simulink model "turbina_viento"  (R2015a)
settings: Solver=ode45  StartTime=0.0  StopTime=50  RelTol=1e-3
libraries: simulink x1
settings Model: Creator=Administrador  LastModifiedBy=Administrador

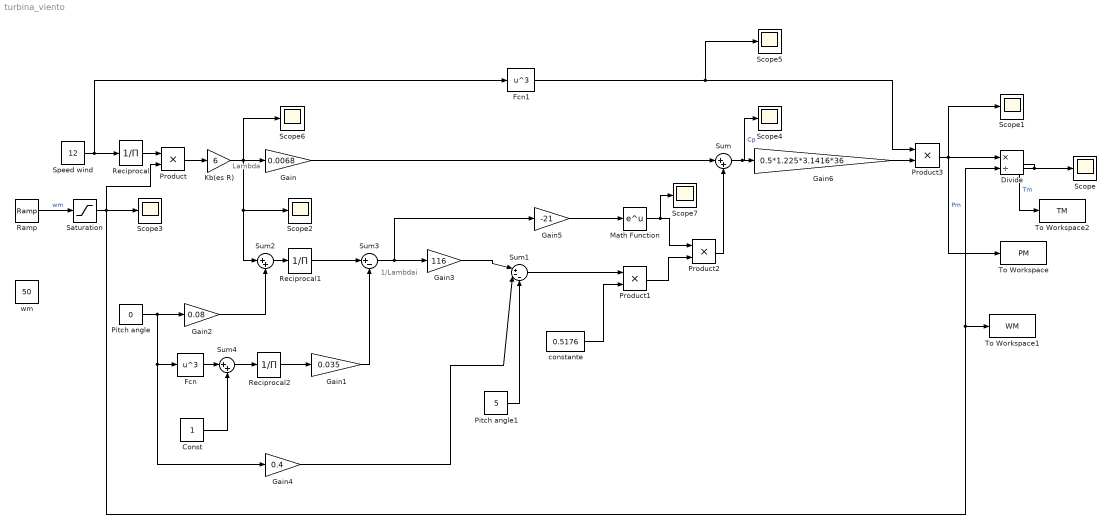
== system turbina_viento ==
  note: 1/Lambdai
  note: Lambda
  Const : Constant
  Divide : Product  Inputs=*/
  Fcn : Fcn  Expr=u^3
  Fcn1 : Fcn  Expr=u^3
  Gain : Gain  Gain=0.0068
  Gain1 : Gain  Gain=0.035
  Gain2 : Gain  Gain=0.08
  Gain3 : Gain  Gain=116
  Gain4 : Gain  Gain=0.4
  Gain5 : Gain  Gain=-21
  Gain6 : Gain  Gain=0.5*1.225*3.1416*36
  Kb(es R) : Gain  Gain=6
  Math Function : Math  SaturateOnIntegerOverflow=on
  Pitch angle : Constant  Value=0
  Pitch angle1 : Constant  Value=5
  Product{,1..3} (4 alike) : Product
  Ramp : simulink/Sources/Ramp  slope=1  start=5  X0=8
  Reciprocal : Product  Inputs=/  SaturateOnIntegerOverflow=on  RndMeth=Zero
  Reciprocal1 : Product  Inputs=/  SaturateOnIntegerOverflow=on  RndMeth=Zero
  Reciprocal2 : Product  Inputs=/  SaturateOnIntegerOverflow=on  RndMeth=Zero
  Saturation : Saturate  UpperLimit=14  LowerLimit=8
  Scope{,1..7} (8 alike) : Scope
      Scope2 settings: SaveName=ScopeData2
      Scope3 settings: SaveName=ScopeData3
      Scope4 settings: SaveName=ScopeData4
      Scope5 settings: SaveName=ScopeData5
      Scope6 settings: SaveName=ScopeData6
      Scope7 settings: SaveName=ScopeData7
  Speed wind : Constant  Value=12
  Sum : Sum  Inputs=|++
  Sum1 : Sum  Inputs=|+--
  Sum2 : Sum  Inputs=|++
  Sum3 : Sum  Inputs=|+-
  Sum4 : Sum  Inputs=|++
  To Workspace : ToWorkspace  VariableName=PM  SaveFormat=Timeseries  SampleTime=-1
  To Workspace1 : ToWorkspace  VariableName=WM  SaveFormat=Timeseries  SampleTime=-1
  To Workspace2 : ToWorkspace  VariableName=TM  SaveFormat=Timeseries  SampleTime=-1
  constante : Constant  Value=0.5176
  wm : Constant  Value=50
  wires:
  Speed wind/1 -> Fcn1/1, Reciprocal/1
  Reciprocal/1 -> Product/1
  Product/1 -> Kb(es R)/1
  Kb(es R)/1 -> Scope6/1, Scope2/1, Sum2/1, Gain/1
  Gain/1 -> Sum/1
  Pitch angle/1 -> Gain2/1, Gain4/1, Fcn/1
  Sum2/1 -> Reciprocal1/1
  Reciprocal1/1 -> Sum3/1
  Gain2/1 -> Sum2/2
  Reciprocal2/1 -> Gain1/1
  Gain1/1 -> Sum3/2
  Fcn/1 -> Sum4/1
  Sum4/1 -> Reciprocal2/1
  Const/1 -> Sum4/2
  Sum3/1 -> Gain5/1, Gain3/1
  Gain3/1 -> Sum1/1
  constante/1 -> Product1/2
  Sum1/1 -> Product1/1
  Gain4/1 -> Sum1/2
  Pitch angle1/1 -> Sum1/3
  Product2/1 -> Sum/2
  Math Function/1 -> Scope7/1, Product2/1
  Product1/1 -> Product2/2
  Gain5/1 -> Math Function/1
  Sum/1 -> Scope4/1, Gain6/1  "Cp"
  Divide/1 -> To Workspace2/1, Scope/1  "Tm"
  Gain6/1 -> Product3/2
  Fcn1/1 -> Scope5/1, Product3/1
  Product3/1 -> To Workspace/1, Scope1/1, Divide/1  "Pm"
  Ramp/1 -> Saturation/1  "wm"
  Saturation/1 -> Product/2, To Workspace1/1, Divide/2, Scope3/1
